simulink model "five"  (R2019b)
settings: Solver=VariableStepAuto  StartTime=0.0  StopTime=10.0  RelTol=1e-3
values from neighbouring files (symbols this model uses):
  i = ii(p)    [fourfun.m]
  j = jj(q)    [fourfun.m]
settings Model: Creator=Pranshu  LastModifiedBy=Pranshu
settings OptimizationCC: BlockReduction=off  DefaultParameterBehavior=Inlined  BufferReuse=off

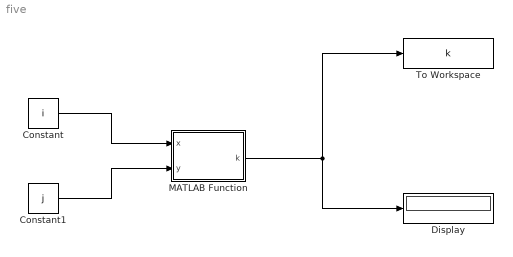
== system five ==
  Constant : Constant  Value=i
  Constant1 : Constant  Value=j
  Display : Display
  MATLAB Function : MATLAB Function  TreatAsAtomicUnit=on
  To Workspace : ToWorkspace  VariableName=k  SampleTime=-1
  wires:
  Constant/1 -> MATLAB Function/1(x)
  Constant1/1 -> MATLAB Function/2(y)
  MATLAB Function/1(k) -> Display/1, To Workspace/1

== matlab function five/MATLAB Function ==
  data: x input; k output; y input
function k = fcn(x, y)

k = x+y;
